simulink model "Lane_Change_Assist"  (R2022b)
settings: configuration reference "CommonModelConfiguration" (kept outside this file)
undefined symbols (not defined in the file): cc_param_145, cc_param_312, LCFG_DSF_Timeout, LCFG_DSF_Timeout2
settings Model: Creator=RPETE142  LastModifiedBy=OTHOMSO1
settings ConfigSetRef: SourceName=CommonModelConfiguration  SourceLocation=Base Workspace

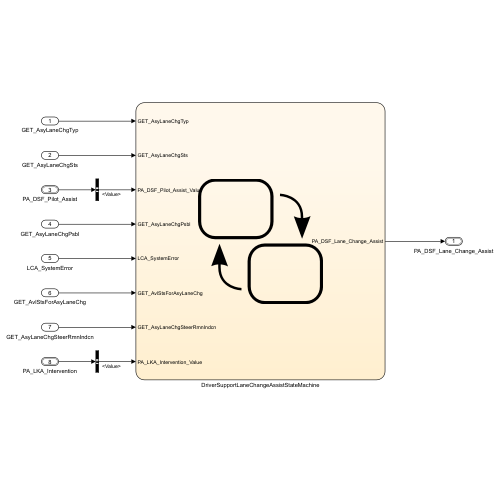
[thumbnail: Simulink's stored preview of the top-level diagram]
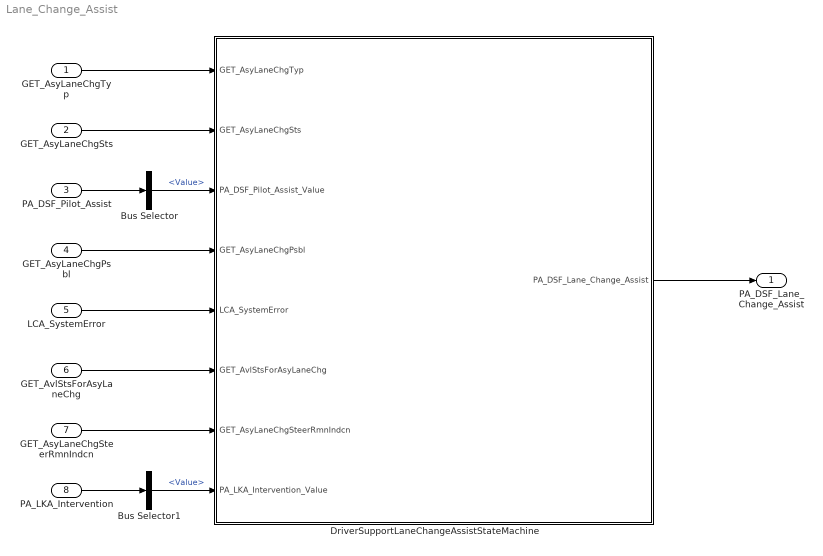
== system Lane_Change_Assist ==
  GET_AsyLaneChgTyp : Inport  OutDataTypeStr=Enum: AsyLaneChgTyp2
  GET_AsyLaneChgSts : Inport  Port=2  OutDataTypeStr=Enum: AsyLaneChgSts2
  PA_DSF_Pilot_Assist : Inport  Port=3  OutDataTypeStr=Bus: PA_DSF
  GET_AsyLaneChgPsbl : Inport  Port=4  OutDataTypeStr=Enum: AsyLaneChgPsbl1
  LCA_SystemError : Inport  Port=5  OutDataTypeStr=boolean
  GET_AvlStsForAsyLaneChg : Inport  Port=6
  GET_AsyLaneChgSteerRmnIndcn : Inport  Port=7  OutDataTypeStr=Enum: OnOff1
  PA_LKA_Intervention : Inport  Port=8  OutDataTypeStr=Bus: StatusAndLKAValue
  Bus Selector : BusSelector  OutputSignals=Value
  Bus Selector1 : BusSelector  OutputSignals=Value
  "DriverSupportLaneChangeAssistStateMachine " : Stateflow chart  TreatAsAtomicUnit=on
  PA_DSF_Lane_Change_Assist : Outport  OutDataTypeStr=Bus: PA_DSF_LCA
  wires:
  GET_AsyLaneChgTyp/1 -> "DriverSupportLaneChangeAssistStateMachine "/1(GET_AsyLaneChgTyp)
  GET_AsyLaneChgSts/1 -> "DriverSupportLaneChangeAssistStateMachine "/2(GET_AsyLaneChgSts)
  PA_DSF_Pilot_Assist/1 -> Bus Selector/1
  Bus Selector/1 -> "DriverSupportLaneChangeAssistStateMachine "/3(PA_DSF_Pilot_Assist_Value)  "<Value>"
  "DriverSupportLaneChangeAssistStateMachine "/1(PA_DSF_Lane_Change_Assist) -> PA_DSF_Lane_Change_Assist/1
  LCA_SystemError/1 -> "DriverSupportLaneChangeAssistStateMachine "/5(LCA_SystemError)
  GET_AsyLaneChgPsbl/1 -> "DriverSupportLaneChangeAssistStateMachine "/4(GET_AsyLaneChgPsbl)
  GET_AvlStsForAsyLaneChg/1 -> "DriverSupportLaneChangeAssistStateMachine "/6(GET_AvlStsForAsyLaneChg)
  GET_AsyLaneChgSteerRmnIndcn/1 -> "DriverSupportLaneChangeAssistStateMachine "/7(GET_AsyLaneChgSteerRmnIndcn)
  PA_LKA_Intervention/1 -> Bus Selector1/1
  Bus Selector1/1 -> "DriverSupportLaneChangeAssistStateMachine "/8(PA_LKA_Intervention_Value)  "<Value>"

== stateflow chart Lane_Change_Assist/DriverSupportLaneChangeAssistStateMachine  ==
  state CARCONFIG_INVALID
    entry:
    PA_DSF_Lane_Change_Assist.Status = E_CommonStatus.NotPresent;
    PA_DSF_Lane_Change_Assist.Value = E_DSF_LCA.LCA_Off;
    PA_DSF_Lane_Change_Assist.Direction = E_Direction.Left;
    PA_DSF_Lane_Change_Assist.Possibility = E_Direction.NoDirection;
    PA_DSF_Lane_Change_Assist.Message = E_DSF_Messages.Messages_Off;
  state SYSTEM_OK
    state intvLKA = isIntervention [function]
      (default) -> (junction 2263)
      (junction 2263) -> (junction 2264) [order 1] : [PA_LKA_Intervention_Value==E_LaneDetection.LKA_Intervention_Left_PA ||...
          | PA_LKA_Intervention_Value==E_LaneDetection.LKA_Intervention_Right_PA ||...
          | PA_LKA_Intervention_Value==E_LaneDetection.LKA_Intervention_Left_PA_China ||...
          | PA_LKA_Intervention_Value==E_LaneDetection.LKA_Intervention_Right_PA_China]
      (junction 2263) -> (junction 2265) [order 2] : {intvLKA = false;}
      (junction 2264) -> (junction 2266) : {intvLKA = true;}
      (junction 2266) -> (junction 2265)
      (junction 2265) -> (junction 2267)
    state isActive = activationCheck [function]
      (default) -> (junction 35)
      (junction 35) -> (junction 28) [order 1] : [PA_DSF_Pilot_Assist_Value==E_DSF_Value.DSF_Active ||...
          | PA_DSF_Pilot_Assist_Value==E_DSF_Value.DSF_Standby]
      (junction 35) -> (junction 29) [order 2] : {isActive = false;}
      (junction 28) -> (junction 30) : {isActive = true;}
      (junction 30) -> (junction 29)
      (junction 29) -> (junction 31)
    state NOT_ACTIVE
      entry:
      PA_DSF_Lane_Change_Assist.Possibility = E_Direction.NoDirection;
      PA_DSF_Lane_Change_Assist.Message = E_DSF_Messages.Messages_Off;
      state HOLD_VALUES
      state FINISH_VALUES
        entry:
        PA_DSF_Lane_Change_Assist.Value =...
        E_DSF_LCA.LCA_Off;
        PA_DSF_Lane_Change_Assist.Status =...
        E_CommonStatus.Disabled;
        PA_DSF_Lane_Change_Assist.Direction =...
        E_Direction.Left;
      (default) -> (junction 2246)
      (junction 2246) -> HOLD_VALUES [order 1] : [PA_DSF_Lane_Change_Assist.Value==...
          | E_DSF_LCA.LCA_Cancelled &&...
          | ~isIntervention]
      (junction 2246) -> FINISH_VALUES [order 2]
      HOLD_VALUES -> (junction 2250) : [after(LCFG_DSF_Timeout2, sec)]
      (junction 2250) -> FINISH_VALUES
    state ACTIVE
      entry:
      PA_DSF_Lane_Change_Assist.Status = E_CommonStatus.Available;
      PA_DSF_Lane_Change_Assist.Message = E_DSF_Messages.Messages_Off;
      state POSSIBILITY [parallel]
        settings: executionOrder=1
        state retVal = checkPossibility [function]
          (default) -> (junction 2080)
          (junction 2080) -> (junction 2079) [order 1] : [GET_AsyLaneChgPsbl == AsyLaneChgPsbl1.AsyLaneChgPsbl1_Le]
              | {PA_DSF_Lane_Change_Assist.Possibility = E_Direction.Left;}
          (junction 2079) -> (junction 2081)
          (junction 2080) -> (junction 2082) [order 2]
          (junction 2082) -> (junction 2081) [order 1] : [GET_AsyLaneChgPsbl == AsyLaneChgPsbl1.AsyLaneChgPsbl1_Ri]
              | {PA_DSF_Lane_Change_Assist.Possibility = E_Direction.Right;}
          (junction 2081) -> (junction 2083)
          (junction 2082) -> (junction 2084) [order 2]
          (junction 2084) -> (junction 2083) [order 1] : [GET_AsyLaneChgPsbl == AsyLaneChgPsbl1.AsyLaneChgPsbl1_Both]
              | {PA_DSF_Lane_Change_Assist.Possibility = E_Direction.BothDirections;}
          (junction 2083) -> (junction 2086) : {retVal = true;}
          (junction 2084) -> (junction 2085) [order 2] : {retVal = false;}
          (junction 2086) -> (junction 2085)
          (junction 2085) -> (junction 2087)
        state IMPOSSIBLE
          entry:
          PA_DSF_Lane_Change_Assist.Possibility = E_Direction.NoDirection;
        state POSSIBLE
        (default) -> IMPOSSIBLE
        IMPOSSIBLE -> POSSIBLE : [checkPossibility]
        POSSIBLE -> IMPOSSIBLE : [~checkPossibility]
      state DIRECTION [parallel]
        settings: executionOrder=2
        state LEFT
          entry:
          PA_DSF_Lane_Change_Assist.Direction =...
          E_Direction.Left;
        state RIGHT
          entry:
          PA_DSF_Lane_Change_Assist.Direction =...
          E_Direction.Right;
        (default) -> (junction 1797)
        (junction 1797) -> (junction 1798) [order 1] : [GET_AsyLaneChgTyp==AsyLaneChgTyp2.AsyLaneChgTyp2_LaneChgRi]
        (junction 1797) -> LEFT [order 2]
        (junction 1798) -> RIGHT
        LEFT -> RIGHT : [GET_AsyLaneChgTyp==...
            | AsyLaneChgTyp2.AsyLaneChgTyp2_LaneChgRi]
        RIGHT -> LEFT : [GET_AsyLaneChgTyp==...
            | AsyLaneChgTyp2.AsyLaneChgTyp2_LaneChgLe]
      state LANE_CHANGE_ASSIST [parallel]
        settings: executionOrder=3
        state ACTIVATED
          entry:
          PA_DSF_Lane_Change_Assist.Value =...
          E_DSF_LCA.LCA_Standby;
          PA_DSF_Lane_Change_Assist.Message =...
          E_DSF_Messages.Messages_Off;
        state EXECUTING
          entry:
          PA_DSF_Lane_Change_Assist.Value =...
          E_DSF_LCA.LCA_Executing;
        state ABORTED_MESSAGE
          entry:
          PA_DSF_Lane_Change_Assist.Value = E_DSF_LCA.LCA_Aborted;
          (default) -> (junction 2205)
          (junction 2205) -> (junction 2206) [order 1] : [GET_AvlStsForAsyLaneChg==...
              | AvlStsForAsyLaneChg.UnavlDueToDrvrAction]
              | {PA_DSF_Lane_Change_Assist.Message =...
              | E_DSF_Messages.Messages_CancelDriverAction;}
          (junction 2205) -> (junction 2216) [order 2]
          (junction 2206) -> (junction 2207)
          (junction 2216) -> (junction 2207) [order 1] : [GET_AvlStsForAsyLaneChg==...
              | AvlStsForAsyLaneChg.UnavlDueToRoadCond]
              | {PA_DSF_Lane_Change_Assist.Message =...
              | E_DSF_Messages.Messages_CancelRoadCondition;}
          (junction 2216) -> (junction 2219) [order 2]
          (junction 2207) -> (junction 2210)
          (junction 2219) -> (junction 2210) [order 1] : [GET_AvlStsForAsyLaneChg==...
              | AvlStsForAsyLaneChg.UnavlDueToSurrndTrffc]
              | {PA_DSF_Lane_Change_Assist.Message =...
              | E_DSF_Messages.Messages_CancelSurroundTraffic;}
          (junction 2219) -> (junction 2221) [order 2]
          (junction 2210) -> (junction 2212)
          (junction 2221) -> (junction 2212) [order 1] : [GET_AvlStsForAsyLaneChg==...
              | AvlStsForAsyLaneChg.UnavlDueToLaneChgCnd]
              | {PA_DSF_Lane_Change_Assist.Message =...
              | E_DSF_Messages.Messages_CancelNoLaneChange;}
          (junction 2221) -> (junction 2223) [order 2]
          (junction 2212) -> (junction 2214)
          (junction 2214) -> (junction 2223)
          (junction 2223) -> (junction 2230)
        state SYSTEM_FAILURE
          entry:
          PA_DSF_Lane_Change_Assist.Value =...
          E_DSF_LCA.LCA_Cancelled;
        (default) -> ACTIVATED
        ACTIVATED -> EXECUTING : %Lane change ongoing
            | [GET_AsyLaneChgSts==...
            | AsyLaneChgSts2.AsyLaneChgSts2_Executing &&...
            | (GET_AsyLaneChgTyp==...
            | AsyLaneChgTyp2.AsyLaneChgTyp2_LaneChgLe ||...
            | GET_AsyLaneChgTyp==...
            | AsyLaneChgTyp2.AsyLaneChgTyp2_LaneChgRi)]
        EXECUTING -> (junction 2168) : %Finished, aborted or failure
            | [GET_AsyLaneChgSts~=...
            | AsyLaneChgSts2.AsyLaneChgSts2_Executing ||...
            | (GET_AsyLaneChgTyp~=...
            | AsyLaneChgTyp2.AsyLaneChgTyp2_LaneChgLe &&...
            | GET_AsyLaneChgTyp~=...
            | AsyLaneChgTyp2.AsyLaneChgTyp2_LaneChgRi)]
        (junction 2168) -> ABORTED_MESSAGE [order 1] : %Lane change aborted
            | [GET_AsyLaneChgSts==...
            | AsyLaneChgSts2.AsyLaneChgSts2_Aborted ||...
            | GET_AsyLaneChgSts==...
            | AsyLaneChgSts2.AsyLaneChgSts2_Ovrdn]
        (junction 2168) -> (junction 2165) [order 2]
        ABORTED_MESSAGE -> (junction 2242) : [after(LCFG_DSF_Timeout, sec) ||...
            | isIntervention]
        (junction 2165) -> ACTIVATED [order 2]
        (junction 2165) -> SYSTEM_FAILURE [order 1] : %System failure
            | [GET_AsyLaneChgTyp==...
            | AsyLaneChgTyp2.AsyLaneChgTyp2_NotAvl ||...
            | GET_AsyLaneChgTyp==...
            | AsyLaneChgTyp2.AsyLaneChgTyp2_SrvRqrd]
        (junction 2238) -> ACTIVATED
        SYSTEM_FAILURE -> (junction 2238) : [after(LCFG_DSF_Timeout, sec) ||...
            | isIntervention]
        (junction 2241) -> (junction 2238)
        (junction 2242) -> (junction 2241)
    (default) -> (junction 1781)
    (junction 1781) -> NOT_ACTIVE [order 2]
    (junction 1781) -> (junction 1782) [order 1] : [activationCheck()]
    NOT_ACTIVE -> ACTIVE : [activationCheck()]
    ACTIVE -> NOT_ACTIVE : [~activationCheck()]
    (junction 1782) -> ACTIVE
  state SYSTEM_ERROR
    entry:
    PA_DSF_Lane_Change_Assist.Status = E_CommonStatus.SystemError;
    PA_DSF_Lane_Change_Assist.Value = E_DSF_LCA.LCA_Off;
    PA_DSF_Lane_Change_Assist.Direction = E_Direction.Left;
    PA_DSF_Lane_Change_Assist.Possibility = E_Direction.NoDirection;
    PA_DSF_Lane_Change_Assist.Message = E_DSF_Messages.Messages_Off;
  (default) -> (junction 284)
  (junction 284) -> CARCONFIG_INVALID [order 2]
  (junction 284) -> (junction 287) [order 1] : %LCA configured
      | [cc_param_312 > 1 ||...
      | cc_param_145 == 4]
  (junction 287) -> SYSTEM_OK [order 2]
  (junction 287) -> (junction 2059) [order 1] : [LCA_SystemError]
  SYSTEM_ERROR -> SYSTEM_OK : [~LCA_SystemError]
  SYSTEM_OK -> SYSTEM_ERROR : [LCA_SystemError]
  (junction 2059) -> SYSTEM_ERROR
  data: intvLKA function_output; isActive function_output; retVal function_output; GET_AsyLaneChgTyp input Enum: AsyLaneChgTyp2; GET_AsyLaneChgSts input Enum: AsyLaneChgSts2; cc_param_312 parameter; cc_param_145 parameter; PA_DSF_Lane_Change_Assist output Bus: PA_DSF_LCA; PA_DSF_Pilot_Assist_Value input Enum: E_DSF_Value; GET_AsyLaneChgPsbl input Enum: AsyLaneChgPsbl1; LCA_SystemError input boolean; GET_AvlStsForAsyLaneChg input Enum: AvlStsForAsyLaneChg; GET_AsyLaneChgSteerRmnIndcn input Enum: OnOff1; PA_LKA_Intervention_Value input Enum: E_LaneDetection; LCFG_DSF_Timeout parameter; LCFG_DSF_Timeout2 parameter
